simulink model "MotionDetection"  (R2020b)
settings: Solver=FixedStepDiscrete  StartTime=0.0  StopTime=54  RelTol=1e-3
undefined symbols (not defined in the file or in its folder): gray, Rec, SDTV
libraries: visionanalysis x2, visionconversions x1, visiongeotforms x1, dspvision x1
settings Model: FPTRunName=Active  ExtModeAutoUpdateStatusClock=off  Creator=The MathWorks, Inc.  LastModifiedBy=carlo
settings DataIOCC: LimitDataPoints=on  SaveFormat=Array  SaveOutput=off  SaveTime=off  ReturnWorkspaceOutputs=off  SignalLoggingName=sigsOut
settings OptimizationCC: ExpressionDepthLimit=2147483647  InitFltsAndDblsToZero=on  EfficientMapNaN2IntZero=off  LifeSpan=inf
settings DebuggingCC: SaveWithParameterizedLinksMsg=none  UnderspecifiedInitializationDetection=Classic  MergeDetectMultiDrivingBlocksExec=none  CheckExecutionContextPreStartOutputMsg=on  CheckExecutionContextRuntimeOutputMsg=on  SignalResolutionControl=TryResolveAllWithWarning  MultiTaskDSMMsg=warning  ParameterPrecisionLossMsg=none  FcnCallInpInsideContextMsg=warning  StateNameClashWarn=warning  SFUnexpectedBacktrackingDiag=warning  SFNoUnconditionalDefaultTransitionDiag=warning  SFExecutionAtInitializationDiag=none  ArithmeticOperatorsInVariantConditions=warning
settings HardwareCC: ProdBitPerPointer=32  ProdBitPerSizeT=32  ProdBitPerPtrDiffT=32  ProdLargestAtomicFloat=None  ProdIntDivRoundTo=Undefined  ProdEndianess=Unspecified  ProdWordSize=32  ProdHWDeviceType=32-bit Generic  TargetBitPerPointer=64  TargetBitPerSizeT=64  TargetBitPerPtrDiffT=64  TargetLongLongMode=on  TargetIntDivRoundTo=Zero  TargetEndianess=LittleEndian  TargetWordSize=64  TargetHWDeviceType=Generic->MATLAB Host Computer  ProdEqTarget=off
settings ModelReferenceCC: PropagateSignalLabelsOutOfModel=off
settings SFSimCC: SimUseLocalCustomCode=off  CustomCodeUndefinedFunction=UseInterfaceOnly
settings RTWCC: RTWUseLocalCustomCode=off
settings CodeAppCC: StateflowObjectComments=on
settings GRTTargetCC: TargetFcnLib=ansi_tfl_tmw.mat  TargetLangStandard=C89/C90 (ANSI)  CombineOutputUpdateFcns=off  GRTInterface=on
settings ConfigComp: CovMetricSettings=dw  CovSaveCumulativeToWorkspaceVar=on  CovSaveSingleToWorkspaceVar=on  CovExternalEMLEnable=off

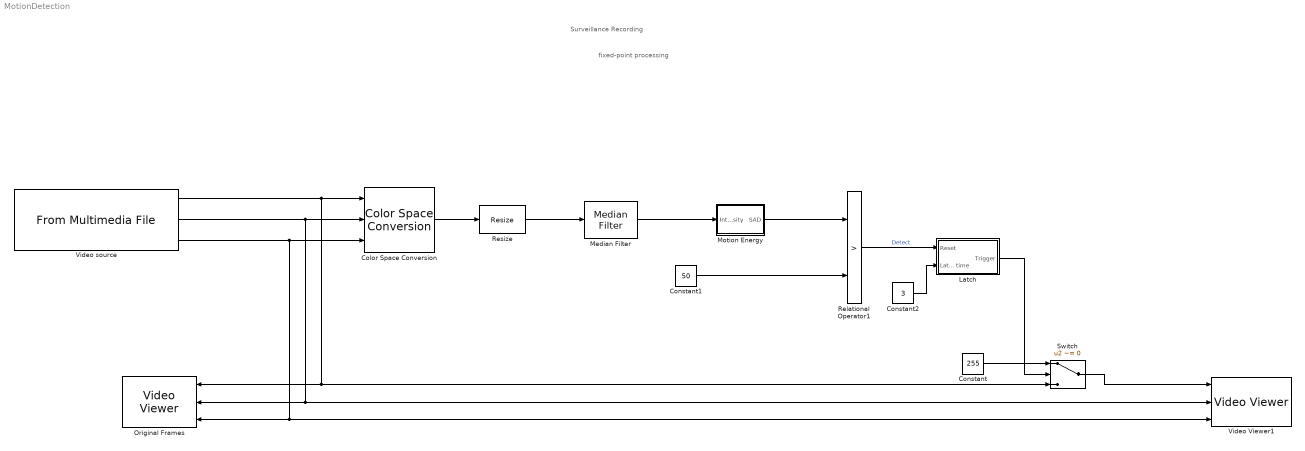
== system MotionDetection ==
  note: Surveillance Recording
  note: fixed-point processing
  Color Space Conversion : visionconversions/Color Space  Conversion  conversion=Obsolete  conversionActive=R'G'B' to intensity  wp_str=D65  rec=Rec. 601 (SDTV)  sys=1125/60/2:1  imagePorts=Separate color signals
  Constant : Constant  Value=255  OutDataTypeStr=uint8
  Constant1 : Constant  Value=50  OutDataTypeStr=Inherit: Inherit via back propagation
  Constant2 : Constant  Value=3  OutDataTypeStr=Inherit: Inherit via back propagation
  Latch : Subsystem
      mask Display: disp('Hold')
  Median Filter : visionanalysis/Median Filter  nghbood=[3 3]  outSize=Same as input port I  padType=Symmetric  padSrc=Specify via dialog  padVal=0  roundingMode=Floor  overflowMode=off
      settings: SourceProductBaseCode=VP
  Motion Energy : Subsystem
  Original Frames : VideoViewer  imagePorts=separate color signals  colormapValue=gray(256)  FigPos=[2 1037 1278 954]  trueSizedOnce=on
  Relational Operator1 : RelationalOperator  Operator=>  OutDataTypeStr=boolean  RndMeth=Nearest  InputSameDT=on
  Resize : visiongeotforms/Resize  specify=Output size as a percentage of input size  rfactor=[25 25]  outCols=25  outRows=25  outRowsCols=[240 320]  interp_method=Bilinear  antialias=on  useROI=off  roiFlag=off  roundingMode=Nearest  overflowMode=on  prodOutputMode=Binary point scaling  prodOutputWordLength=32  prodOutputFracLength=10
      settings: SourceProductBaseCode=VP
  Switch : Switch  Criteria=u2 ~= 0  Threshold=1
  Video Viewer1 : VideoViewer  imagePorts=separate color signals  colormapValue=gray(256)  FigPos=[1282 1037 1278 929]
  Video source : dspvision/From Multimedia File  inputFilename=D:\3DPrints\Motion_Detection_Camera\VideosRossana\190923_PS\Canon\190923_Canon_PA_visitas.mp4  readRange=[1 Inf]  loop=on  numPlays=inf  outputStreams=Video only  videoDataType=uint8  audioDataType=int16  inheritSampleTime=on  userDefinedSampleTime=0.1  noAudioOutput=off  isIntensityVideo=off  fourcc=RGB  colorVideoFormat=Separate color signals  outputEOF=off  dataOrg=Column-major  audioFrameSize=1024  computeAudioFrameSize=off  outSamplingMode=Frame based
  wires:
  Constant1/1 -> Relational Operator1/2
  Video source/2 -> Video Viewer1/2, Original Frames/2, Color Space Conversion/2
  Video source/3 -> Original Frames/3, Video Viewer1/3, Color Space Conversion/3
  Constant/1 -> Switch/1
  Video source/1 -> Switch/3, Original Frames/1, Color Space Conversion/1
  Switch/1 -> Video Viewer1/1
  Color Space Conversion/1 -> Resize/1
  Resize/1 -> Median Filter/1
  Motion Energy/1(SAD) -> Relational Operator1/1
  Median Filter/1 -> Motion Energy/1(Intensity)
  Relational Operator1/1 -> Latch/1(Reset)  "Detect"
  Latch/1(Trigger) -> Switch/2
  Constant2/1 -> Latch/2(Latch time)

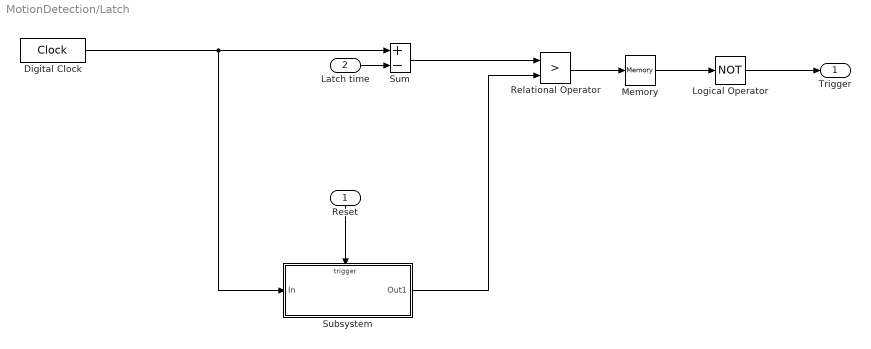
== system MotionDetection/Latch ==
  Reset : Inport
  Latch time : Inport  Port=2
  Digital Clock : DigitalClock  SampleTime=-1
  Logical Operator : Logic  Operator=NOT  Inputs=1
  Memory : Memory  InitialCondition=1
  Relational Operator : RelationalOperator  Operator=>  RndMeth=Nearest  InputSameDT=on
  Subsystem : Subsystem
  Sum : Sum  Inputs=+-  InputSameDT=on  SaturateOnIntegerOverflow=on  OutDataTypeStr=Inherit: Same as first input
  Trigger : Outport  InitialOutput=0  VectorParamsAs1DForOutWhenUnconnected=off
  wires:
  Reset/1 -> Subsystem/Trigger
  Sum/1 -> Relational Operator/1
  Subsystem/1(Out1) -> Relational Operator/2
  Relational Operator/1 -> Memory/1
  Memory/1 -> Logical Operator/1
  Logical Operator/1 -> Trigger/1
  Latch time/1 -> Sum/2
  Digital Clock/1 -> Subsystem/1(In), Sum/1

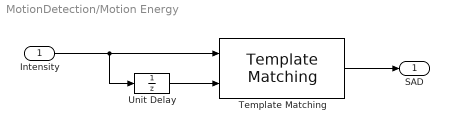
== system MotionDetection/Motion Energy ==
  Intensity : Inport
  Template Matching : visionanalysis/Template Matching  metric=Maximum absolute difference  output=Metric matrix  method=Exhaustive  nMetric=off  nSize=3  roi=off  roiValid=off  roundingMode=Floor  overflowMode=on  prodOutputMode=Binary point scaling  prodOutputWordLength=32  prodOutputFracLength=0
      settings: SourceProductBaseCode=VP
  Unit Delay : UnitDelay  SampleTime=-1  HasFrameUpgradeWarning=on
  SAD : Outport  VectorParamsAs1DForOutWhenUnconnected=off
  wires:
  Template Matching/1 -> SAD/1
  Intensity/1 -> Template Matching/1, Unit Delay/1
  Unit Delay/1 -> Template Matching/2

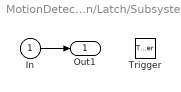
== system MotionDetection/Latch/Subsystem ==
  In : Inport
  Trigger : TriggerPort  TriggerType=either  VariantControl=Variant
  Out1 : Outport  InitialOutput=-10  VectorParamsAs1DForOutWhenUnconnected=off
  wires:
  In/1 -> Out1/1
